simulink model "furuta_pendulum_final"  (R2014a)
settings: Solver=ode45  StartTime=0.0  StopTime=10  RelTol=1e-3
values from neighbouring files (symbols this model uses):
  K = acker(A,B,P)    [Ackermann_Furuta_Pendulum_TEC_Final.m]    (also in Furuta_Pendulum.m; Furuta_Pendulum_Final.m = lqr(A,B,Q,R); Planta.m = lqr(A,B,Q,R); Planta2.m = lqr(A,B,Q,R))
  X1 = -m*r*g/J    (= -46.8065899705)    [Ackermann_Furuta_Pendulum_TEC_Final.m]    (also in Furuta_Pendulum_Final.m; Furuta_Pendulum_TEC_Variante.m = -16.1262627486; Planta.m = -16.1262627486; Planta2.m)
  X2 = -(Ke^2)/(J*R)    (= -180.497257309)    [Ackermann_Furuta_Pendulum_TEC_Final.m]    (also in Furuta_Pendulum_Final.m; Furuta_Pendulum_TEC_Variante.m = 978.093147544; Planta.m = 978.093147544; Planta2.m)
  X3 = Ke/(J*R)    (= 173.931851703)    [Ackermann_Furuta_Pendulum_TEC_Final.m]    (also in Furuta_Pendulum_Final.m; Planta2.m)
  Y1 = g*(J+m*r^2)/(J*l)    (= 135.38817428)    [Ackermann_Furuta_Pendulum_TEC_Final.m]    (also in Furuta_Pendulum_Final.m; Furuta_Pendulum_TEC_Variante.m = 46.64525386; Planta.m = 46.64525386; Planta2.m)
  Y2 = (r*(Ke^2))/(J*R*l)    (= 268.306733838)    [Ackermann_Furuta_Pendulum_TEC_Final.m]    (also in Furuta_Pendulum_Final.m; Furuta_Pendulum_TEC_Variante.m = -755.366987922; Planta.m = -755.366987922; Planta2.m)
  Y3 = -(Ke*r)/(J*R*l)    (= -258.547347126)    [Ackermann_Furuta_Pendulum_TEC_Final.m]    (also in Furuta_Pendulum_Final.m; Planta2.m)
libraries: simulink_extras x1
settings Model: Creator=Juan Rojas  LastModifiedBy=Juan Rojas

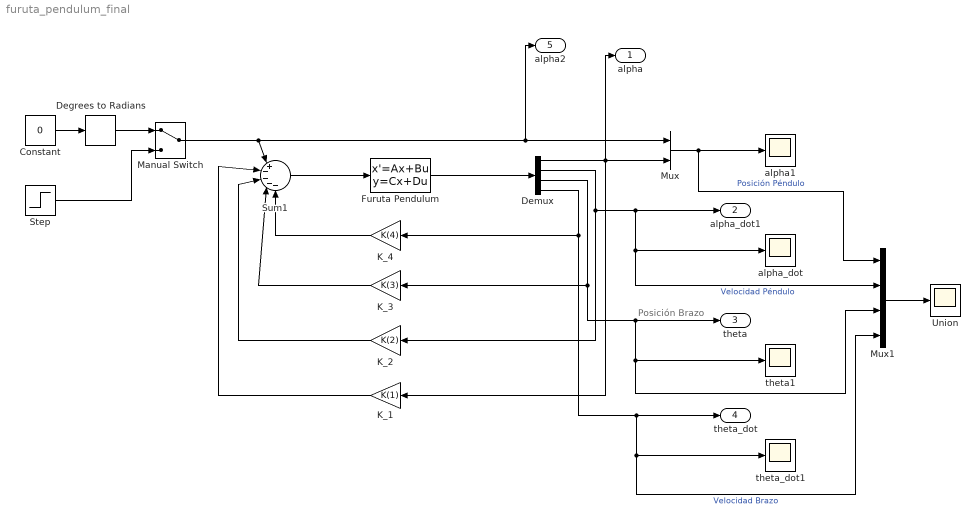
== system furuta_pendulum_final ==
  note: Posición Brazo
  Constant : Constant  Value=0
  Degrees to Radians : simulink_extras/Transformations/Degrees to Radians
  Demux : Demux
  Furuta Pendulum : StateSpace  A="[0 0 1 0;   0 0 0 1;   0 X1 X2 0;   0 Y1 Y2 0]"  B=[0;0;X3;Y3]  C=eye(4)  D=[0;0;0;0]  X0=[0.1*pi/180;0;0;0]
  K_1 : Gain  Gain=K(1)
  K_2 : Gain  Gain=K(2)
  K_3 : Gain  Gain=K(3)
  K_4 : Gain  Gain=K(4)
  Manual Switch : ManualSwitch
  Mux : Mux  Inputs=2
  Mux1 : Mux
  Step : Step  Before=1*pi/180  After=0*pi/180  SampleTime=0
  Sum1 : Sum  Inputs=|+----
  "Union " : Scope
      settings: ShowLegends=on  YMin=-1  YMax=1  SaveName=ScopeData4
  alpha1 : Scope
  alpha_dot : Scope
  theta1 : Scope
      settings: SaveName=ScopeData2
  theta_dot1 : Scope
      settings: SaveName=ScopeData3
  alpha : Outport
  alpha_dot1 : Outport  Port=2
  theta : Outport  Port=3
  theta_dot : Outport  Port=4
  alpha2 : Outport  Port=5
  wires:
  Manual Switch/1 -> Sum1/1, Mux/1, alpha2/1
  Furuta Pendulum/1 -> Demux/1
  Sum1/1 -> Furuta Pendulum/1
  Demux/1 -> Mux/2, alpha/1, K_1/1
  Demux/4 -> K_4/1, theta_dot/1, theta_dot1/1, Mux1/4  "Velocidad Brazo"
  Mux1/1 -> "Union "/1
  Mux/1 -> Mux1/1, alpha1/1  "Posición Péndulo"
  Demux/2 -> alpha_dot1/1, Mux1/2, alpha_dot/1, K_2/1  "Velocidad Péndulo"
  Demux/3 -> K_3/1, theta/1, theta1/1, Mux1/3
  Constant/1 -> Degrees to Radians/1
  Degrees to Radians/1 -> Manual Switch/1
  K_1/1 -> Sum1/2
  K_2/1 -> Sum1/3
  K_3/1 -> Sum1/4
  K_4/1 -> Sum1/5
  Step/1 -> Manual Switch/2
